simulink model "controller"  (R2020a)
settings: Solver=VariableStepAuto  StartTime=0.0  StopTime=10.0  RelTol=1e-3
values from neighbouring files (symbols this model uses):
  Ki = 200    [data_in_workspace.mat]    (also in motor_data.sldd = 200.0)
  Kp = 300    [data_in_workspace.mat]    (also in motor_data.sldd = 100.0)
  Ts = 0.02    [data_in_workspace.mat]    (also in motor_data.sldd = 0.01)
settings Model: Creator=shweta  LastModifiedBy=shweta
settings DataIOCC: SaveOutput=off  SaveTime=off
settings DebuggingCC: ModelReferenceExtraNoncontSigs=none

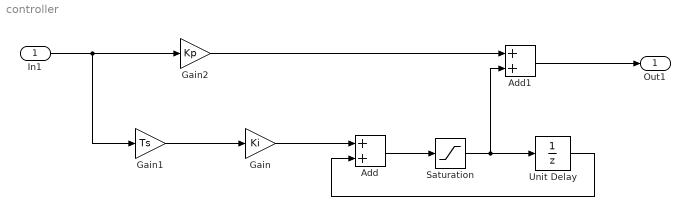
== system controller ==
  In1 : Inport  OutDataTypeStr=double  PortDimensions=1  SampleTime=0
  Add : Sum
  Add1 : Sum
  Gain : Gain  Gain=Ki
  Gain1 : Gain  Gain=Ts
  Gain2 : Gain  Gain=Kp
  Saturation : Saturate  UpperLimit=1  LowerLimit=-1
  Unit Delay : UnitDelay  SampleTime=-1  HasFrameUpgradeWarning=on
  Out1 : Outport  OutDataTypeStr=double  PortDimensions=1  SampleTime=0
  wires:
  Gain/1 -> Add/1
  Add/1 -> Saturation/1
  Unit Delay/1 -> Add/2
  In1/1 -> Gain2/1, Gain1/1
  Add1/1 -> Out1/1
  Gain2/1 -> Add1/1
  Gain1/1 -> Gain/1
  Saturation/1 -> Add1/2, Unit Delay/1
